simulink subsystem "Autopilot"  (R2021b)
settings: Solver=VariableStepAuto  StartTime=0.0  StopTime=10.0  RelTol=1e-3
libraries: simulink_extras x3, slpidlib x1
settings Model: Creator=janbe  LastModifiedBy=vojtech.voska

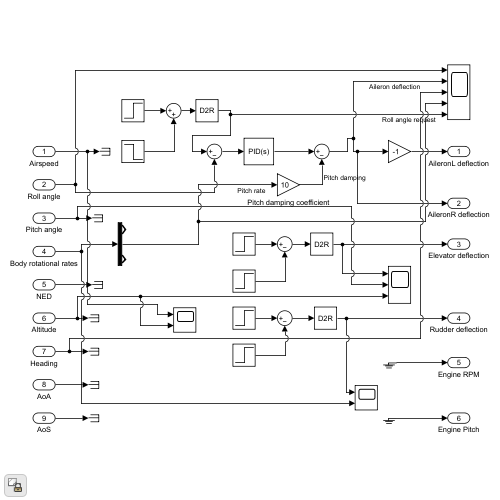
[thumbnail: Simulink's stored preview of the top-level diagram]
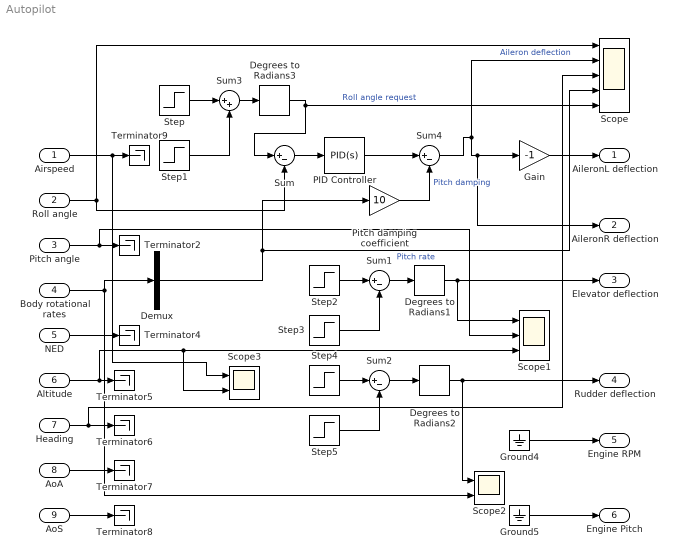
== system Autopilot ==
  Airspeed : Inport  Unit=m/s
  Roll angle : Inport  Port=2  Unit=rad
  Pitch angle : Inport  Port=3  Unit=rad
  Body rotational rates : Inport  Port=4  Unit=rad/s
  NED : Inport  Port=5  Unit=m
  Altitude : Inport  Port=6  Unit=m
  Heading : Inport  Port=7  Unit=rad
  AoA : Inport  Port=8  Unit=rad
  AoS : Inport  Port=9  Unit=rad
  Degrees to Radians1 : simulink_extras/Transformations/Degrees to Radians
  Degrees to Radians2 : simulink_extras/Transformations/Degrees to Radians
  Degrees to Radians3 : simulink_extras/Transformations/Degrees to Radians
  Demux : Demux  Outputs=3
  Gain : Gain  Gain=-1
  Ground4 : Ground
  Ground5 : Ground
  PID Controller : slpidlib/PID Controller  Controller=PID  Form=Parallel  TimeDomain=Continuous-time  UseExternalTs=off  SampleTime=-1  IntegratorMethod=Forward Euler  FilterMethod=Forward Euler  ControllerParametersSource=internal  P=5  I=2  D=0  UseFilter=on  N=3.61035899502078  TunerSelectOption=Transfer Function Based (PID Tuner App)  InitialConditionSource=internal  InitialConditionForIntegrator=0  InitialConditionForFilter=0  DifferentiatorICPrevScaledInput=0  ExternalReset=none  TrackingMode=off  Kt=1  LimitOutput=off  SatLimitsSource=internal  UpperSaturationLimit=inf  LowerSaturationLimit=-inf  LinearizeAsGain=on  AntiWindupMode=none  Kb=1  POutMin=[]  POutMax=[]  IOutMin=[]  IOutMax=[]  DOutMin=[]  DOutMax=[]  NOutMin=[]  NOutMax=[]  SumOutMin=[]  SumOutMax=[]  SaturationOutMin=[]  SaturationOutMax=[]  PParamMin=[]  PParamMax=[]  IParamMin=[]  IParamMax=[]  DParamMin=[]  DParamMax=[]  NParamMin=[]  NParamMax=[]  KbParamMin=[]  KbParamMax=[]  KtParamMin=[]  KtParamMax=[]  KbOutMin=[]  KbOutMax=[]  KtOutMin=[]  KtOutMax=[]  IntegratorOutMin=[]  IntegratorOutMax=[]  FilterOutMin=[]  FilterOutMax=[]  SumI1OutMin=[]  SumI1OutMax=[]  SumI2OutMin=[]  SumI2OutMax=[]  SumI3OutMin=[]  SumI3OutMax=[]  SumI4OutMin=[]  SumI4OutMax=[]  SumDOutMin=[]  SumDOutMax=[]  DifferentiatorOutMin=[]  DifferentiatorOutMax=[]  FilterDiffOutCoefMin=[]  FilterDiffOutCoefMax=[]  ReciprocalOutMin=[]  ReciprocalOutMax=[]  SumDenOutMin=[]  SumDenOutMax=[]  SumNumOutMin=[]  SumNumOutMax=[]  DivideOutMin=[]  DivideOutMax=[]  UdiffTsProdOutMin=[]  UdiffTsProdOutMax=[]  NTsProdOutMin=[]  NTsProdOutMax=[]  UintegralTsProdOutMin=[]  UintegralTsProdOutMax=[]  UngainTsProdOutMin=[]  UngainTsProdOutMax=[]  IntegratorContinuousStateAttributes=''  IntegratorStateMustResolveToSignalObject=off  IntegratorRTWStateStorageClass=Auto  FilterContinuousStateAttributes=''  FilterStateMustResolveToSignalObject=off  FilterRTWStateStorageClass=Auto  ParallelPVariant=InternalParameters  IdealPVariant=Disabled  IVariant=InternalParameters  DVariant=InternalParameters  IntegratorVariant=Continuous  SatVariant=Disabled  AWVariant=Passthrough  PCopyVariant=Disabled  TRVariant=Disabled  FdbkBlocksVariant=Forward  IdealPFdbkVariant=Disabled  SatFdbkVariant=Disabled  DerivativeFilterVariant=ContFilter  NVariant=InternalParameters  NCopyVariant=Disabled  FilterICVariant=InternalICsFilter  IntegratorICVariant=InternalICs  ExternalResetVariant=Disabled  TRSumVariant=Passthrough  SumFdbkVariant=Disabled  SumVariant=Sum_PID  TsampFilterVariant=InternalTs  TsampNgainVariant=Passthrough  TsampIntegralVariant=Passthrough  ExternalSaturationOutDataTypeStr=Inherit: Same as second input
  Pitch damping coefficient : Gain  Gain=10
  Scope : Scope  NumInputPorts=5
  Scope1 : Scope  NumInputPorts=3
  Scope2 : Scope  NumInputPorts=2
  Scope3 : Scope  NumInputPorts=2
  Step : Step  Time=10  After=5  SampleTime=0
  Step1 : Step  Time=15  After=-5  SampleTime=0
  Step2 : Step  Time=100  SampleTime=0
  Step3 : Step  Time=110  SampleTime=0
  Step4 : Step  Time=150  SampleTime=0
  Step5 : Step  Time=160  SampleTime=0
  Sum{,1..2,4} (4 alike) : Sum  Inputs=|+-
  Sum3 : Sum  Inputs=|++
  Terminator{2,4..9} (7 alike) : Terminator
  AileronL deflection : Outport  Unit=rad
  AileronR deflection : Outport  Port=2  Unit=rad
  Elevator deflection : Outport  Port=3  Unit=rad
  Rudder deflection : Outport  Port=4  Unit=rad
  Engine RPM : Outport  Port=5  Unit=rpm  PortDimensions=[2,1]
  Engine Pitch : Outport  Port=6  Unit=deg  PortDimensions=[2,1]
  wires:
  Airspeed/1 -> Terminator9/1, Scope3/1
  Pitch angle/1 -> Terminator2/1, Scope1/2
  Body rotational rates/1 -> Scope2/2, Demux/1
  NED/1 -> Terminator4/1
  Altitude/1 -> Terminator5/1, Scope1/3, Scope3/2
  Heading/1 -> Scope/3, Terminator6/1
  AoA/1 -> Terminator7/1
  AoS/1 -> Terminator8/1
  Sum4/1 -> Scope/2, Gain/1, AileronR deflection/1  "Aileron deflection"
  Sum2/1 -> Degrees to Radians2/1
  Ground4/1 -> Engine RPM/1
  Ground5/1 -> Engine Pitch/1
  Step3/1 -> Sum1/2
  Step2/1 -> Sum1/1
  Step5/1 -> Sum2/2
  Step4/1 -> Sum2/1
  Sum1/1 -> Degrees to Radians1/1
  Degrees to Radians1/1 -> Scope1/1, Elevator deflection/1
  Degrees to Radians2/1 -> Rudder deflection/1, Scope2/1
  Sum/1 -> PID Controller/1
  Step/1 -> Sum3/1
  Step1/1 -> Sum3/2
  Sum3/1 -> Degrees to Radians3/1
  Roll angle/1 -> Scope/1, Sum/2
  Degrees to Radians3/1 -> Scope/5, Sum/1  "Roll angle request"
  Gain/1 -> AileronL deflection/1
  Demux/2 -> Scope/4, Pitch damping coefficient/1  "Pitch rate"
  Pitch damping coefficient/1 -> Sum4/2  "Pitch damping"
  PID Controller/1 -> Sum4/1
